simulink model "second_order_DDPG_sin"  (R2021a)
settings: Solver=FixedStepAuto  StartTime=0.0  StopTime=500  FixedStep=0.001  RelTol=1e-3
libraries: rllib x1, simulink x1
settings Model: Creator=Steven  LastModifiedBy=德尔菲神庙

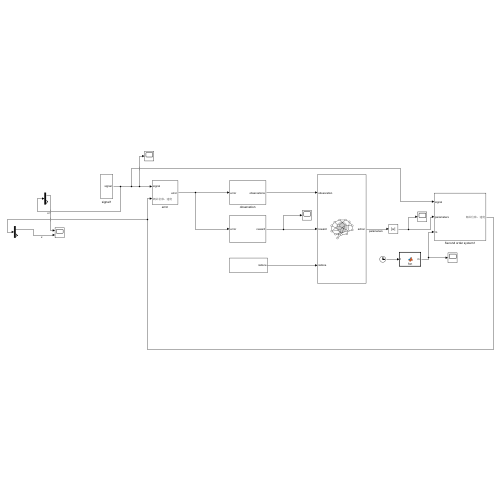
[thumbnail: Simulink's stored preview of the top-level diagram]
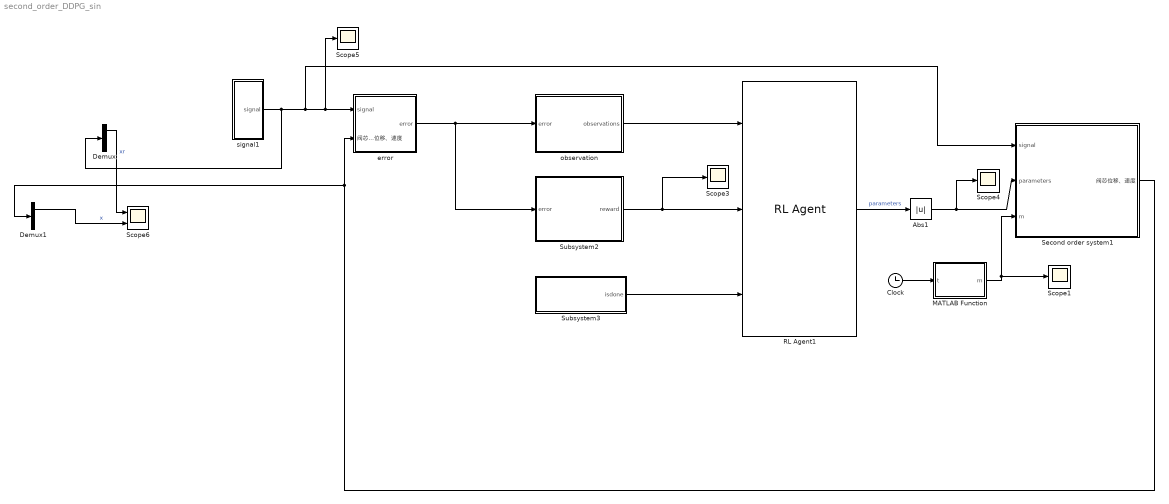
== system second_order_DDPG_sin ==
  Abs1 : Abs
  Clock : Clock
  Demux : Demux  Outputs=2
  Demux1 : Demux  Outputs=2
  MATLAB Function : MATLAB Function  TreatAsAtomicUnit=on
  RL Agent1 : rllib/RL Agent  Agent=agent_second_order_Trained_4_17_finished  ExternalActionAsInput=off  ProvideLastAction=off  ProvideCumRwd=off  TreatAsDirectFeedthrough=on  UseStrictObservationDataTypes=off
  Scope{1,3..5} (4 alike) : Scope
  Scope6 : Scope  NumInputPorts=2
  Second order system1 : Subsystem
  Subsystem2 : Subsystem
  Subsystem3 : Subsystem
  error : Subsystem
  observation : Subsystem
  signal1 : Subsystem
  wires:
  Second order system1/1(阀芯位移、速度) -> Demux1/1, error/2(阀芯位移、速度)
  Subsystem3/1(isdone) -> RL Agent1/3
  observation/1(observations) -> RL Agent1/1
  RL Agent1/1 -> Abs1/1  "parameters"
  signal1/1(signal) -> Demux/1, Second order system1/1(signal), Scope5/1, error/1(signal)
  error/1(error) -> Subsystem2/1(error), observation/1(error)
  Abs1/1 -> Scope4/1, Second order system1/2(parameters)
  Demux/1 -> Scope6/1  "xr"
  Demux1/1 -> Scope6/2  "x"
  MATLAB Function/1(m) -> Second order system1/3(m), Scope1/1
  Clock/1 -> MATLAB Function/1(t)
  Subsystem2/1(reward) -> Scope3/1, RL Agent1/2

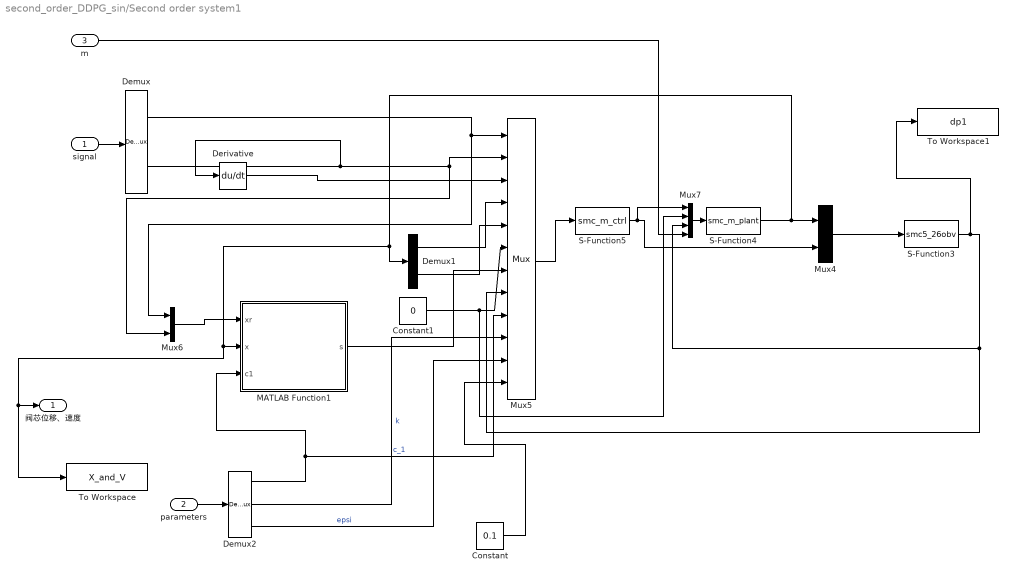
== system second_order_DDPG_sin/Second order system1 ==
  signal : Inport
  parameters : Inport  Port=2
  m : Inport  Port=3
  Constant : Constant  Value=0.1
  Constant1 : Constant  Value=0
  Demux : Demux  Outputs=2
  Demux1 : Demux  Outputs=2
  Demux2 : Demux  Outputs=3
  Derivative : Derivative
  MATLAB Function1 : MATLAB Function  TreatAsAtomicUnit=on
  Mux4 : Mux  Inputs=2
  Mux5 : Mux  Inputs=12
  Mux6 : Mux  Inputs=2
  Mux7 : Mux
  S-Function3 : S-Function  FunctionName=smc5_26obv  SFunctionDeploymentMode=off  EnableBusSupport=off
  S-Function4 : S-Function  FunctionName=smc_m_plant  SFunctionDeploymentMode=off  EnableBusSupport=off
  S-Function5 : S-Function  FunctionName=smc_m_ctrl  SFunctionDeploymentMode=off  EnableBusSupport=off
  To Workspace : ToWorkspace  VariableName=X_and_V  SampleTime=-1
  To Workspace1 : ToWorkspace  VariableName=dp1  SampleTime=-1
      settings: Save2DSignal=2-D array (concatenate along first dimension)
  阀芯位移、速度 : Outport
  wires:
  S-Function3/1 -> To Workspace1/1, Mux7/3, Mux5/8
  Mux5/1 -> S-Function5/1
  Constant1/1 -> Mux7/2, Mux5/6
  MATLAB Function1/1(s) -> Mux5/7
  Demux1/2 -> Mux5/5
  S-Function4/1 -> Demux1/1, To Workspace/1, 阀芯位移、速度/1, MATLAB Function1/2(x), Mux4/1
  Mux4/1 -> S-Function3/1
  Mux6/1 -> MATLAB Function1/1(xr)
  Demux/1 -> Mux6/1, Mux5/1
  Demux1/1 -> Mux5/4
  Mux7/1 -> S-Function4/1
  S-Function5/1 -> Mux7/1, Mux4/2
  signal/1 -> Demux/1
  Demux/2 -> Mux6/2, Mux5/2, Derivative/1
  parameters/1 -> Demux2/1
  Demux2/1 -> MATLAB Function1/3(c1), Mux5/9  "c_1"
  Demux2/2 -> Mux5/10  "k"
  Demux2/3 -> Mux5/11  "epsi"
  Derivative/1 -> Mux5/3
  m/1 -> Mux7/4
  Constant/1 -> Mux5/12

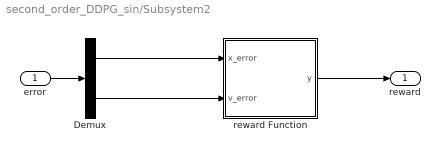
== system second_order_DDPG_sin/Subsystem2 ==
  error : Inport
  Demux : Demux  Outputs=2
  reward Function : MATLAB Function  TreatAsAtomicUnit=on
  reward : Outport
  wires:
  error/1 -> Demux/1
  Demux/1 -> reward Function/1(x_error)
  Demux/2 -> reward Function/2(v_error)
  reward Function/1(y) -> reward/1

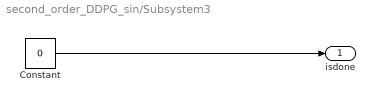
== system second_order_DDPG_sin/Subsystem3 ==
  Constant : Constant  Value=0
  isdone : Outport
  wires:
  Constant/1 -> isdone/1

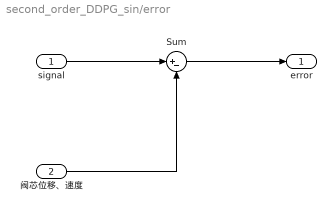
== system second_order_DDPG_sin/error ==
  signal : Inport
  阀芯位移、速度 : Inport  Port=2
  Sum : Sum  Inputs=|+-
  error : Outport
  wires:
  signal/1 -> Sum/1
  阀芯位移、速度/1 -> Sum/2
  Sum/1 -> error/1

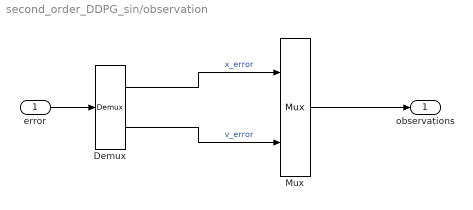
== system second_order_DDPG_sin/observation ==
  error : Inport
  Demux : Demux  Outputs=2
  Mux : Mux  Inputs=2
  observations : Outport
  wires:
  Mux/1 -> observations/1
  error/1 -> Demux/1
  Demux/1 -> Mux/1  "x_error"
  Demux/2 -> Mux/2  "v_error"

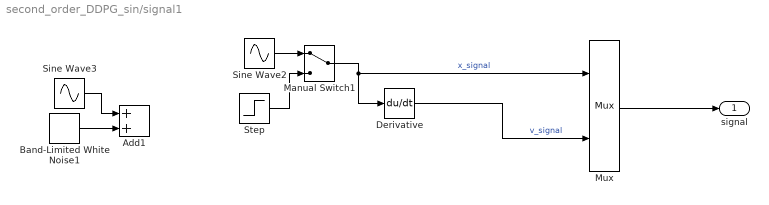
== system second_order_DDPG_sin/signal1 ==
  Add1 : Sum
  Band-Limited White Noise1 : simulink/Sources/Band-Limited White Noise  Cov=[1e-5*1e-5*0.1]  Ts=0.1  seed=[0]
  Derivative : Derivative
  Manual Switch1 : ManualSwitch
  Mux : Mux  Inputs=2
  Sine Wave2 : Sin  Amplitude=1e-3  Frequency=1*pi  SampleTime=0
  Sine Wave3 : Sin  Amplitude=1e-4  Frequency=30*pi  SampleTime=0
  Step : Step  Time=0  After=1e-4  SampleTime=0
  signal : Outport
  wires:
  Sine Wave2/1 -> Manual Switch1/1
  Step/1 -> Manual Switch1/2
  Manual Switch1/1 -> Mux/1, Derivative/1  "x_signal"
  Derivative/1 -> Mux/2  "v_signal"
  Mux/1 -> signal/1
  Band-Limited White Noise1/1 -> Add1/2
  Sine Wave3/1 -> Add1/1

== matlab function second_order_DDPG_sin/Second order system1/MATLAB Function1 ==
  data: xr input; s output; x input; c1 input
function s = S(xr,x,c1)
s = c1*(xr(1)-x(1)) + (xr(2)-x(2));

== matlab function second_order_DDPG_sin/Subsystem2/reward Function ==
  data: x_error input; y output; v_error input
function y = fcn(x_error,v_error)
y = -x_error*20000000-v_error*100;

== matlab function second_order_DDPG_sin/MATLAB Function ==
  data: t input; m output
function m = fcn(t)
% fcn - 计算质量m随时间t变化的函数
%   t - 时间，单位秒

% 初始化参数
initial_mass = 0.1; % 初始质量
final_mass = 0.05;  % 最终质量
start_decay_time = 10; % 开始衰减的时间，单位秒
decay_duration = 5;    % 衰减持续时间，单位秒

% 计算质量
if t < start_decay_time
    m = initial_mass;
% elseif t < start_decay_time + decay_duration
%     % 线性衰减
%     m = initial_mass - (initial_mass - final_mass) * ((t - start_decay_time) / decay_duration);
else
    m = final_mass;
end
end
